simulink model "lab1_model_est"  (R2024b)
settings: Solver=ode45  StartTime=0.0  StopTime=sIn.time  RelTol=1e-3
undefined symbols (not defined in the file or in its folder): degs2rpm, drv, filt, gbox, mld, mot, PID, rads2rpm, rpm2degs, sens, sIn
libraries: simulink_extras x3, simulink x3
settings Model: Creator=pries  LastModifiedBy=pries
settings DataIOCC: ReturnWorkspaceOutputs=off

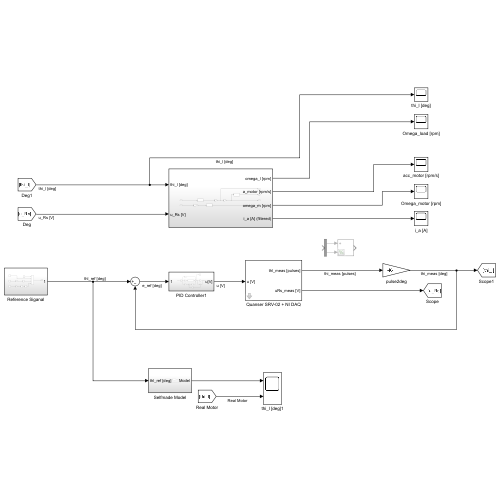
[thumbnail: Simulink's stored preview of the top-level diagram]
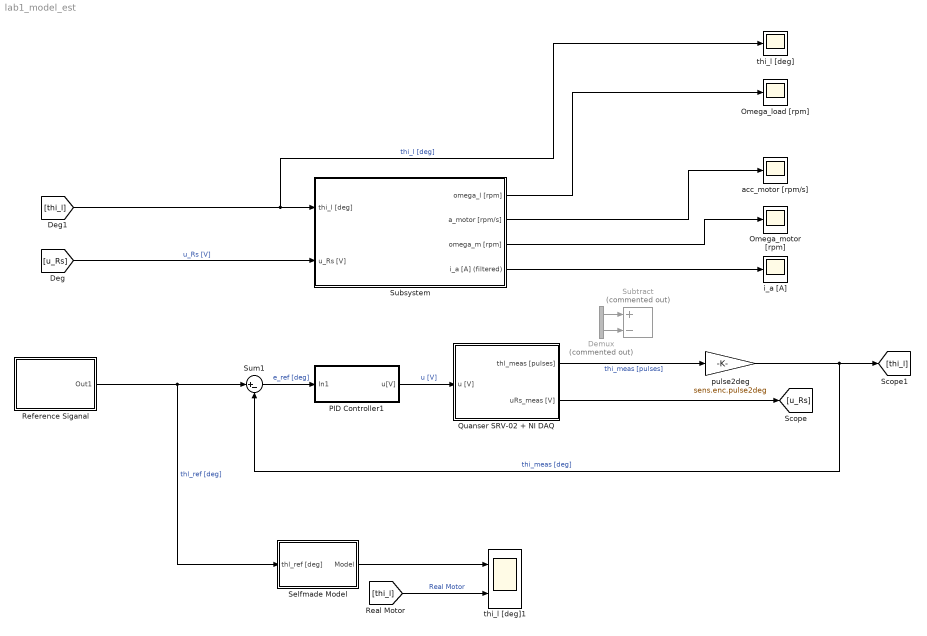
== system lab1_model_est ==
  Demux : Demux  Commented=on  Outputs=2
  Omega_load [rpm] : Scope
  Omega_motor [rpm] : Scope
  PID Controller1 : Subsystem
  Quanser SRV-02 + NI DAQ : Subsystem  mask(Quanser SRV-02 (with inertial load) + NI DAQ){Ts=0.001, fricType=Coulomb + viscous}
      mask prompts: Ts "NI DAQ Sample Time:"; fricType "Friction model"
      mask help: Quanser SRV-02 (with inertial load) + NI DAQ model.
      mask init:
      | %%  Sensors data
      | 
      | %   shunt resistor
      | sens.curr.Rs = 0.5;                         %   resistance [Ohm]   
      | sens.curr.uRs_std = 0.01;                   %   voltage noise standard dev [V]                           
      | sens.curr.uRs_var = sens.curr.uRs_std^2;	%   voltage noise variance [V^2]
      | 
      | %   Hewlett-Packard HEDS-5540#A06 optical encoder
      | sens.enc.ppr = 500*4;                       %   pulses per rotation
      | sens.enc.pulse2deg = 360/sens.enc.ppr;      %   [pulses] -> [deg]
      | sens.enc.pulse2rad = 2*pi/sens.enc.ppr;     %   [pulses] -> [rad]
      | sens.enc.deg2pulse = sens.enc.ppr/360;      %   [deg] -> [pulses]
      | sens.enc.rad2pulse = sens.enc.ppr/2/pi;     %   [rad] -> [pulses]
      | 
      | 
      | %%  Data acquisition board (daq) data
      | 
      | %   NI PCI-6221 DAC data
      | daq.dac.bits = 16;                                  %   resolution (bits)
      | daq.dac.fs   = 10;                                  %   full scale 
      | daq.dac.q    = 2*daq.dac.fs/(2^daq.dac.bits-1);     %	quantization
      | 
      | %   NI PCI-6221 ADC data
      | daq.adc.bits = 16;                                  %   resolution (bits)
      | daq.adc.fs   = 10;                                  %   full scale (as set in SLDRT Analog Input block)
      | daq.adc.q    = 2*daq.adc.fs/(2^daq.adc.bits-1);     %   quantization
      mask Help:
      | Riccardo Antonello (antonello@dei.unipd.it)
      | 
      | April 24, 2020
      | 
      | Dept. of Information Engineering, University of Padova
      mask TypeOptions fricType: Coulomb + viscous | Karnopp
  Reference Siganal : Subsystem
  Selfmade Model : Subsystem
  Subsystem : Subsystem
  Subtract : Sum  Commented=on  Inputs=+-
  Sum1 : Sum  Inputs=|+-
  acc_motor [rpm/s] : Scope
  i_a [A] : Scope
  pulse2deg : Gain  Gain=sens.enc.pulse2deg
  thi_l [deg] : Scope
  thi_l [deg]1 : Scope  NumInputPorts=2
  wires:
  Quanser SRV-02 + NI DAQ/1(thl_meas [pulses]) -> pulse2deg/1  "thi_meas [pulses]"
  Sum1/1 -> PID Controller1/1(In1)  "e_ref [deg]"
  pulse2deg/1 -> Sum1/2, [thi_l]  "thi_meas [deg]"
  Quanser SRV-02 + NI DAQ/2(uRs_meas [V]) -> [u_Rs]
  [thi_l] -> thi_l [deg]/1, Subsystem/1(thi_l [deg])  "thi_l [deg]"
  PID Controller1/1(u[V]) -> Quanser SRV-02 + NI DAQ/1(u [V])  "u [V]"
  [u_Rs] -> Subsystem/2(u_Rs [V])  "u_Rs [V]"
  Subsystem/1(omega_l [rpm]) -> Omega_load [rpm]/1
  Subsystem/2(a_motor [rpm/s]) -> acc_motor [rpm/s]/1
  Subsystem/3(omega_m [rpm]) -> Omega_motor [rpm]/1
  Subsystem/4(i_a [A] (filtered)) -> i_a [A]/1
  Demux/1 -> Subtract/1
  Demux/2 -> Subtract/2
  Reference Siganal/1(Out1) -> Selfmade Model/1(thl_ref [deg]), Sum1/1  "thl_ref [deg]"
  Selfmade Model/1(Model) -> thi_l [deg]1/1
  [thi_l] -> thi_l [deg]1/2  "Real Motor"

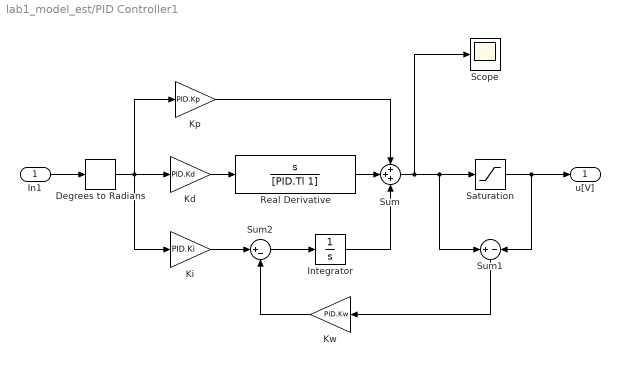
== system lab1_model_est/PID Controller1 ==
  In1 : Inport
  Degrees to Radians : simulink_extras/Transformations/Degrees to Radians
  Integrator : Integrator
  Kd : Gain  Gain=PID.Kd
  Ki : Gain  Gain=PID.Ki
  Kp : Gain  Gain=PID.Kp
  Kw : Gain  Gain=PID.Kw
  Real Derivative : TransferFcn  Numerator=[1 0]  Denominator=[PID.Tl 1]
  Saturation : Saturate  UpperLimit=10  LowerLimit=-10
  Scope : Scope
  Sum : Sum  Inputs=+++
  Sum1 : Sum  Inputs=+|-
  Sum2 : Sum  Inputs=|+-
  u[V] : Outport
  wires:
  In1/1 -> Degrees to Radians/1
  Sum/1 -> Scope/1, Sum1/1, Saturation/1
  Saturation/1 -> Sum1/2, u[V]/1
  Degrees to Radians/1 -> Ki/1, Kd/1, Kp/1
  Kd/1 -> Real Derivative/1
  Integrator/1 -> Sum/3
  Kp/1 -> Sum/1
  Real Derivative/1 -> Sum/2
  Ki/1 -> Sum2/1
  Sum2/1 -> Integrator/1
  Kw/1 -> Sum2/2
  Sum1/1 -> Kw/1

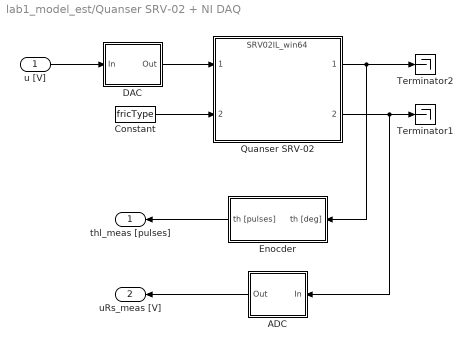
== system lab1_model_est/Quanser SRV-02 + NI DAQ ==
  u [V] : Inport
  ADC : Subsystem
  Constant : Constant  Value=fricType
  DAC : Subsystem
  Enocder : Subsystem
  Quanser SRV-02 : ModelReference  ModelNameDialog=SRV02IL_win64.slxp  ModelReferenceVersion=1.44  CopyOfModelProtected=on
  Terminator1 : Terminator
  Terminator2 : Terminator
  thl_meas [pulses] : Outport
  uRs_meas [V] : Outport  Port=2
  wires:
  Constant/1 -> Quanser SRV-02/2
  Quanser SRV-02/1 -> Terminator2/1, Enocder/1(th [deg])
  u [V]/1 -> DAC/1(In)
  Quanser SRV-02/2 -> Terminator1/1, ADC/1(In)
  DAC/1(Out) -> Quanser SRV-02/1
  ADC/1(Out) -> uRs_meas [V]/1
  Enocder/1(th [pulses]) -> thl_meas [pulses]/1

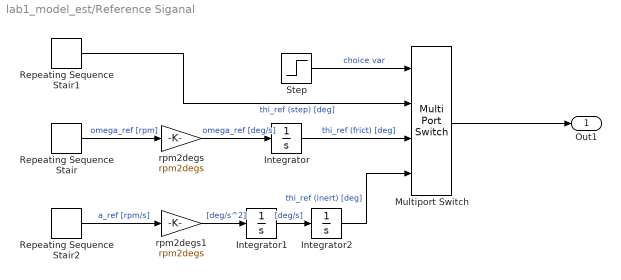
== system lab1_model_est/Reference Siganal ==
  Integrator : Integrator
  Integrator1 : Integrator
  Integrator2 : Integrator
  Multiport Switch : MultiPortSwitch  SaturateOnIntegerOverflow=off  InputSameDT=off
  Repeating Sequence Stair : simulink/Sources/Repeating Sequence Stair  OutValues=frict_est.ref  tsamp=frict_est.time  OutMin=[]  OutMax=[]  OutDataTypeStr=double  OutputDataTypeScalingMode=double  OutDataType=fixdt(0,8)  ConRadixGroup=Best Precision: Vector-wise  OutScaling=2^-12
  Repeating Sequence Stair1 : simulink/Sources/Repeating Sequence Stair  OutValues=step_resp.ref  tsamp=step_resp.time  OutMin=[]  OutMax=[]  OutDataTypeStr=double  OutputDataTypeScalingMode=double  OutDataType=fixdt(0,8)  ConRadixGroup=Best Precision: Vector-wise  OutScaling=2^-12
  Repeating Sequence Stair2 : simulink/Sources/Repeating Sequence Stair  OutValues=inert_est.ref  tsamp=inert_est.time  OutMin=[]  OutMax=[]  OutDataTypeStr=double  OutputDataTypeScalingMode=double  OutDataType=fixdt(0,8)  ConRadixGroup=Best Precision: Vector-wise  OutScaling=2^-12
  Step : Step  Time=0  After=sIn.program  SampleTime=0
  rpm2degs : Gain  Gain=rpm2degs
  rpm2degs1 : Gain  Gain=rpm2degs
  Out1 : Outport
  wires:
  Integrator2/1 -> Multiport Switch/4  "thi_ref (inert) [deg]"
  Integrator1/1 -> Integrator2/1  "[deg/s]"
  rpm2degs/1 -> Integrator/1  "omega_ref [deg/s]"
  Repeating Sequence Stair1/1 -> Multiport Switch/2  "thi_ref (step) [deg]"
  Integrator/1 -> Multiport Switch/3  "thi_ref (frict) [deg]"
  Repeating Sequence Stair2/1 -> rpm2degs1/1  "a_ref [rpm/s]"
  rpm2degs1/1 -> Integrator1/1  "[deg/s^2]"
  Step/1 -> Multiport Switch/1  "choice var"
  Repeating Sequence Stair/1 -> rpm2degs/1  "omega_ref [rpm]"
  Multiport Switch/1 -> Out1/1

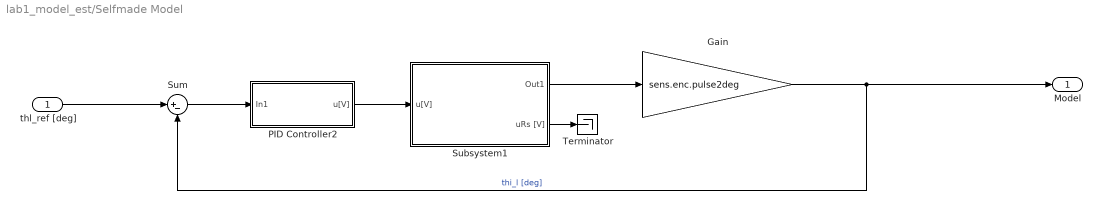
== system lab1_model_est/Selfmade Model ==
  thl_ref [deg] : Inport
  Gain : Gain  Gain=sens.enc.pulse2deg
  PID Controller2 : Subsystem
  Subsystem1 : Subsystem
  Sum : Sum  Inputs=|+-
  Terminator : Terminator
  Model : Outport
  wires:
  thl_ref [deg]/1 -> Sum/1
  Subsystem1/1(Out1) -> Gain/1
  Subsystem1/2(uRs [V]) -> Terminator/1
  PID Controller2/1(u[V]) -> Subsystem1/1(u[V])
  Sum/1 -> PID Controller2/1(In1)
  Gain/1 -> Model/1, Sum/2  "thi_l [deg]"

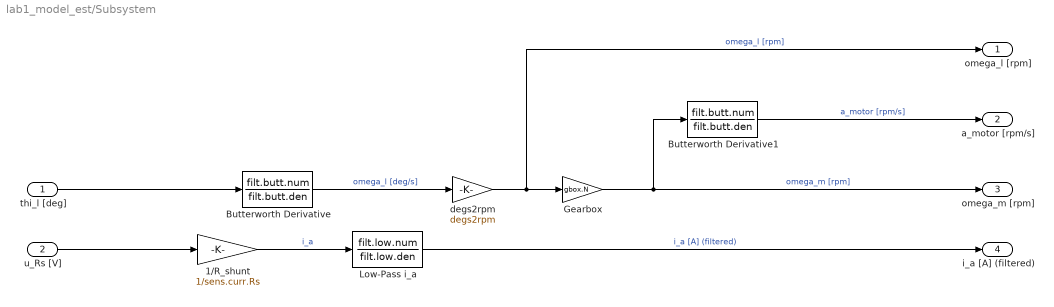
== system lab1_model_est/Subsystem ==
  thi_l [deg] : Inport
  u_Rs [V] : Inport  Port=2
  1/R_shunt : Gain  Gain=1/sens.curr.Rs
  Butterworth Derivative : TransferFcn  Numerator=filt.butt.num  Denominator=filt.butt.den
  Butterworth Derivative1 : TransferFcn  Numerator=filt.butt.num  Denominator=filt.butt.den
  Gearbox : Gain  Gain=gbox.N
  Low-Pass i_a : TransferFcn  Numerator=filt.low.num  Denominator=filt.low.den
  degs2rpm : Gain  Gain=degs2rpm
  omega_l [rpm] : Outport
  a_motor [rpm/s] : Outport  Port=2
  omega_m [rpm] : Outport  Port=3
  i_a [A] (filtered) : Outport  Port=4
  wires:
  Gearbox/1 -> omega_m [rpm]/1, Butterworth Derivative1/1  "omega_m [rpm]"
  u_Rs [V]/1 -> 1/R_shunt/1
  degs2rpm/1 -> omega_l [rpm]/1, Gearbox/1  "omega_l [rpm]"
  thi_l [deg]/1 -> Butterworth Derivative/1
  Low-Pass i_a/1 -> i_a [A] (filtered)/1  "i_a [A] (filtered)"
  Butterworth Derivative/1 -> degs2rpm/1  "omega_l [deg/s]"
  1/R_shunt/1 -> Low-Pass i_a/1  "i_a"
  Butterworth Derivative1/1 -> a_motor [rpm/s]/1  "a_motor [rpm/s]"

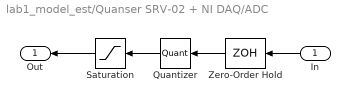
== system lab1_model_est/Quanser SRV-02 + NI DAQ/ADC ==
  In : Inport
  Quantizer : Quantizer  QuantizationInterval=daq.adc.q
  Saturation : Saturate  UpperLimit=daq.adc.fs  LowerLimit=-daq.adc.fs
  Zero-Order Hold : ZeroOrderHold  SampleTime=Ts
  Out : Outport
  wires:
  Zero-Order Hold/1 -> Quantizer/1
  Quantizer/1 -> Saturation/1
  In/1 -> Zero-Order Hold/1
  Saturation/1 -> Out/1

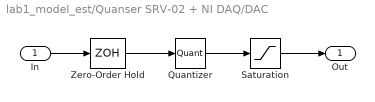
== system lab1_model_est/Quanser SRV-02 + NI DAQ/DAC ==
  In : Inport
  Quantizer : Quantizer  QuantizationInterval=daq.dac.q
  Saturation : Saturate  UpperLimit=daq.dac.fs  LowerLimit=-daq.dac.fs
  Zero-Order Hold : ZeroOrderHold  SampleTime=Ts
  Out : Outport
  wires:
  Saturation/1 -> Out/1
  Zero-Order Hold/1 -> Quantizer/1
  In/1 -> Zero-Order Hold/1
  Quantizer/1 -> Saturation/1

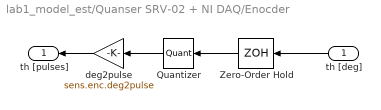
== system lab1_model_est/Quanser SRV-02 + NI DAQ/Enocder ==
  th [deg] : Inport
  Quantizer : Quantizer  QuantizationInterval=sens.enc.pulse2deg
  Zero-Order Hold : ZeroOrderHold  SampleTime=Ts
  deg2pulse : Gain  Gain=sens.enc.deg2pulse
  th [pulses] : Outport
  wires:
  deg2pulse/1 -> th [pulses]/1
  Zero-Order Hold/1 -> Quantizer/1
  th [deg]/1 -> Zero-Order Hold/1
  Quantizer/1 -> deg2pulse/1

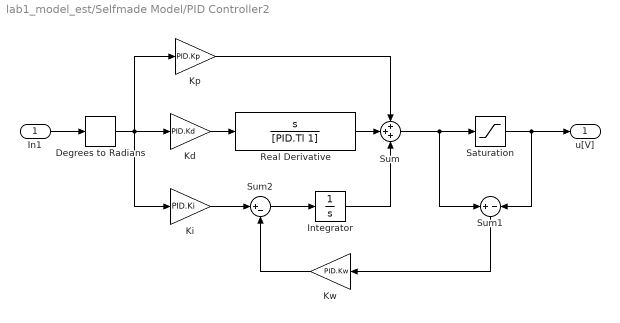
== system lab1_model_est/Selfmade Model/PID Controller2 ==
  In1 : Inport
  Degrees to Radians : simulink_extras/Transformations/Degrees to Radians
  Integrator : Integrator
  Kd : Gain  Gain=PID.Kd
  Ki : Gain  Gain=PID.Ki
  Kp : Gain  Gain=PID.Kp
  Kw : Gain  Gain=PID.Kw
  Real Derivative : TransferFcn  Numerator=[1 0]  Denominator=[PID.Tl 1]
  Saturation : Saturate  UpperLimit=10  LowerLimit=-10
  Sum : Sum  Inputs=+++
  Sum1 : Sum  Inputs=+|-
  Sum2 : Sum  Inputs=|+-
  u[V] : Outport
  wires:
  In1/1 -> Degrees to Radians/1
  Sum/1 -> Sum1/1, Saturation/1
  Saturation/1 -> Sum1/2, u[V]/1
  Degrees to Radians/1 -> Ki/1, Kd/1, Kp/1
  Kd/1 -> Real Derivative/1
  Integrator/1 -> Sum/3
  Kp/1 -> Sum/1
  Real Derivative/1 -> Sum/2
  Ki/1 -> Sum2/1
  Sum2/1 -> Integrator/1
  Kw/1 -> Sum2/2
  Sum1/1 -> Kw/1

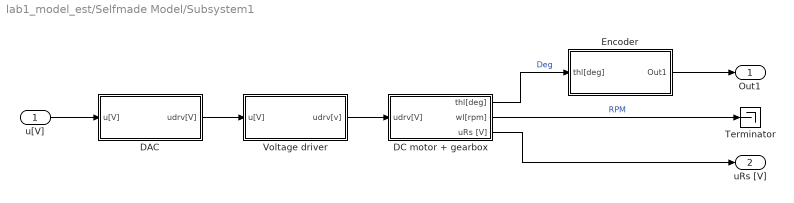
== system lab1_model_est/Selfmade Model/Subsystem1 ==
  u[V] : Inport
  DAC : Subsystem
  DC motor + gearbox : Subsystem
  Encoder : Subsystem
  Terminator : Terminator
  Voltage driver : Subsystem
  Out1 : Outport
  uRs [V] : Outport  Port=2
  wires:
  DC motor + gearbox/1(thl[deg]) -> Encoder/1(thl[deg])  "Deg"
  u[V]/1 -> DAC/1(u[V])
  DC motor + gearbox/2(wl[rpm]) -> Terminator/1  "RPM"
  DAC/1(udrv[V]) -> Voltage driver/1(u[V])
  Voltage driver/1(udrv[v]) -> DC motor + gearbox/1(udrv[V])
  Encoder/1(Out1) -> Out1/1
  DC motor + gearbox/3(uRs [V]) -> uRs [V]/1

== system lab1_model_est/Selfmade Model/Subsystem1/DAC ==
  u[V] : Inport
  Quantizer : Quantizer  QuantizationInterval=daq.dac.q
  Saturation : Saturate  UpperLimit=10  LowerLimit=-10
  Zero-Order Hold : ZeroOrderHold  SampleTime=1e-3
  udrv[V] : Outport
  wires:
  Zero-Order Hold/1 -> Quantizer/1
  u[V]/1 -> Zero-Order Hold/1
  Quantizer/1 -> Saturation/1
  Saturation/1 -> udrv[V]/1

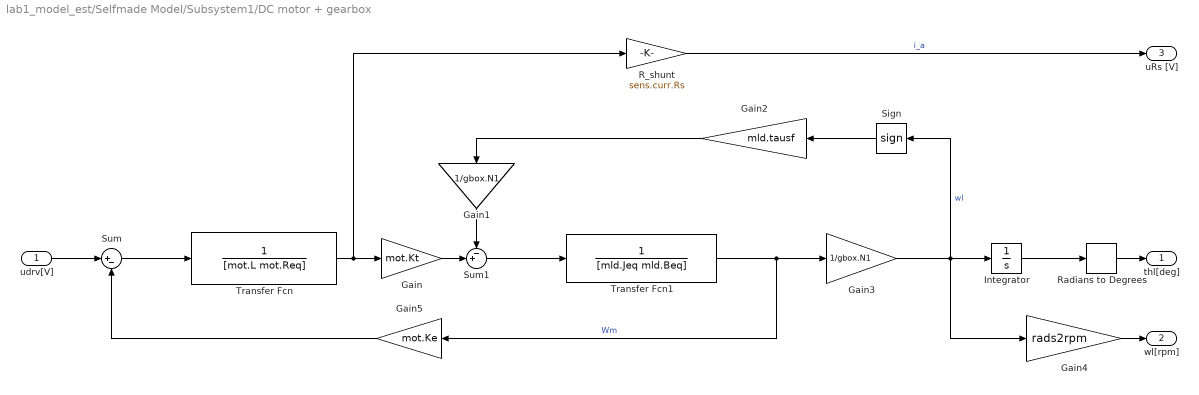
== system lab1_model_est/Selfmade Model/Subsystem1/DC motor + gearbox ==
  udrv[V] : Inport
  Gain : Gain  Gain=mot.Kt
  Gain1 : Gain  Gain=1/gbox.N1
  Gain2 : Gain  Gain=mld.tausf
  Gain3 : Gain  Gain=1/gbox.N1
  Gain4 : Gain  Gain=rads2rpm
  Gain5 : Gain  Gain=mot.Ke
  Integrator : Integrator
  R_shunt : Gain  Gain=sens.curr.Rs
  Radians to Degrees : simulink_extras/Transformations/Radians to Degrees
  Sign : Signum  ZeroCross=off
  Sum : Sum  Inputs=|+-
  Sum1 : Sum  Inputs=-+|
  Transfer Fcn : TransferFcn  Denominator=[mot.L mot.Req]
  Transfer Fcn1 : TransferFcn  Denominator=[mld.Jeq mld.Beq]
  thl[deg] : Outport
  wl[rpm] : Outport  Port=2
  uRs [V] : Outport  Port=3
  wires:
  udrv[V]/1 -> Sum/1
  Sum/1 -> Transfer Fcn/1
  Transfer Fcn/1 -> R_shunt/1, Gain/1
  Gain1/1 -> Sum1/1
  Gain2/1 -> Gain1/1
  Sign/1 -> Gain2/1
  Transfer Fcn1/1 -> Gain5/1, Gain3/1  "Wm"
  Gain3/1 -> Gain4/1, Sign/1, Integrator/1  "wl"
  Integrator/1 -> Radians to Degrees/1
  Radians to Degrees/1 -> thl[deg]/1
  Gain4/1 -> wl[rpm]/1
  Sum1/1 -> Transfer Fcn1/1
  Gain/1 -> Sum1/2
  Gain5/1 -> Sum/2
  R_shunt/1 -> uRs [V]/1  "i_a"

== system lab1_model_est/Selfmade Model/Subsystem1/Encoder ==
  thl[deg] : Inport
  Gain : Gain  Gain=1/sens.enc.pulse2deg
  Quantizer : Quantizer  QuantizationInterval=sens.enc.pulse2deg
  Zero-Order Hold : ZeroOrderHold  SampleTime=1e-3
  Out1 : Outport
  wires:
  thl[deg]/1 -> Zero-Order Hold/1
  Gain/1 -> Out1/1
  Quantizer/1 -> Gain/1
  Zero-Order Hold/1 -> Quantizer/1

== system lab1_model_est/Selfmade Model/Subsystem1/Voltage driver ==
  u[V] : Inport
  Saturation : Saturate  UpperLimit=12  LowerLimit=-12
  Transfer Fcn : TransferFcn  Numerator=[drv.dcgain]  Denominator=[drv.Tc 1]
  udrv[v] : Outport
  wires:
  u[V]/1 -> Transfer Fcn/1
  Transfer Fcn/1 -> Saturation/1
  Saturation/1 -> udrv[v]/1
